simulink model "ModelAVRs"  (Simulink 10.0)
settings: Solver=VariableStepAuto  StartTime=0.0  StopTime=10.0  RelTol=1e-3
settings Model: Creator=Donny  LastModifiedBy=Donny
settings DataIOCC: SaveFormat=Dataset  ReturnWorkspaceOutputs=on
settings OptimizationCC: LifeSpan=auto
settings DebuggingCC: UnderspecifiedInitializationDetection=Simplified  MergeDetectMultiDrivingBlocksExec=error  SFUnexpectedBacktrackingDiag=error  SFNoUnconditionalDefaultTransitionDiag=error  SFExecutionAtInitializationDiag=warning  ArithmeticOperatorsInVariantConditions=error
settings HardwareCC: ProdBitPerPointer=64  ProdBitPerSizeT=64  ProdBitPerPtrDiffT=64  ProdLargestAtomicFloat=Float  ProdIntDivRoundTo=Zero  ProdEndianess=LittleEndian  ProdWordSize=64  ProdHWDeviceType=Intel->x86-64 (Windows64)
settings ModelReferenceCC: PropagateSignalLabelsOutOfModel=on
settings SFSimCC: SimUseLocalCustomCode=on  CustomCodeUndefinedFunction=FilterOut
settings RTWCC: RTWUseLocalCustomCode=on
settings CodeAppCC: StateflowObjectComments=off
settings GRTTargetCC: TargetLangStandard=C99 (ISO)  CombineOutputUpdateFcns=on  GRTInterface=off
settings ConfigComp: CovMetricSettings=dwe  CovHtmlReporting=off  CovSaveCumulativeToWorkspaceVar=off  CovSaveSingleToWorkspaceVar=off

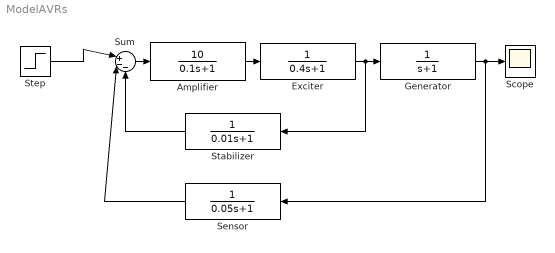
== system ModelAVRs ==
  Amplifier : TransferFcn  Numerator=[10]  Denominator=[0.1 1]
  Exciter : TransferFcn  Denominator=[0.4 1]
  Generator : TransferFcn  Denominator=[1 1]
  Scope : Scope
  Sensor : TransferFcn  Denominator=[0.05 1]
  Stabilizer : TransferFcn  Denominator=[0.01 1]
  Step : Step  SampleTime=0
  Sum : Sum  Inputs=|+--
  wires:
  Amplifier/1 -> Exciter/1
  Sum/1 -> Amplifier/1
  Exciter/1 -> Stabilizer/1, Generator/1
  Stabilizer/1 -> Sum/3
  Sensor/1 -> Sum/2
  Step/1 -> Sum/1
  Generator/1 -> Sensor/1, Scope/1
